simulink model "satellite_dynamics"  (R2025a)
settings: Solver=ode4  StartTime=0.0  StopTime=5400* 5  FixedStep=gyro.Ts  RelTol=1e-6
values from neighbouring files (symbols this model uses):
  altitude = 279e3    (= 279000)    [orbit_params.m]
  G = 6.674e-11    [orbit_params.m]    (also in update_MEKF_new.m = [-eye(3,3), zeros(3,3),zeros(3,3);          zeros(3,3), eye(; update_MEKF_old.m = [-eye(3,3), zeros(3,3);          zeros(3,3), eye(3,3)]; wheel_analysis.m = [ D)
  h_default = h_default + wheel.omega_initial(f) *  wheel.I_II * wheel.axes(:,f)    [orbit_params.m]
  K = convhulln(V)    [wheel_analysis.m]
  m = size(A, 2)    [wheel_analysis.m]
  omega_icrf2b_initial = [-0.3804;-0.2976;0.06] *0    [orbit_params.m]
  P_initial = blkdiag(eye(3) * gyro.sigma_v^2 * 1e4 ,eye(3) * gyro.sigma_u^2 * 1e5)    [orbit_params.m]
  Q_c = blkdiag(eye(3) * gyro.sigma_v^2/2 ,eye(3) * gyro.sigma_u^2/2 )    [orbit_params.m]
  q_icrf2b_initial = q_icrf2b_initial/norm(q_icrf2b_initial)    [orbit_params.m]
  q_initial = q_icrf2b_initial    [orbit_params.m]
  R_k_star = blkdiag(star.sigma_cross^2,star.sigma_cross^2,star.sigma_bore^2) * ((1/3600) * pi/180)^2    [orbit_params.m]
  r_offset = [1;1;5] * 1e-2    [orbit_params.m]
  regulation_kp = regulation.kp    [orbit_params.m]
  s = sign(h_bias)    [min_h.m]
  Ts = 0.1    [orbit_params.m]    (also in untitled2.m = 0.005)
  x_initial = zeros(6,1)    [orbit_params.m]
undefined symbols (not defined in the file or in its folder): DiscIntNeverNeededParam, earth, gyro, Kalman, mag, mag_torque, NEO, regulation, star, sun, tracking, wheel
libraries: utilities x24, simulink_extras x21, aerolibutil x20, dspmathops x19, matrix_library x9, simulink x8, dspstat3 x8, sharedutil x3, aerolibgravity2 x1, eeGeneralControl x1
(part 2 of 2)

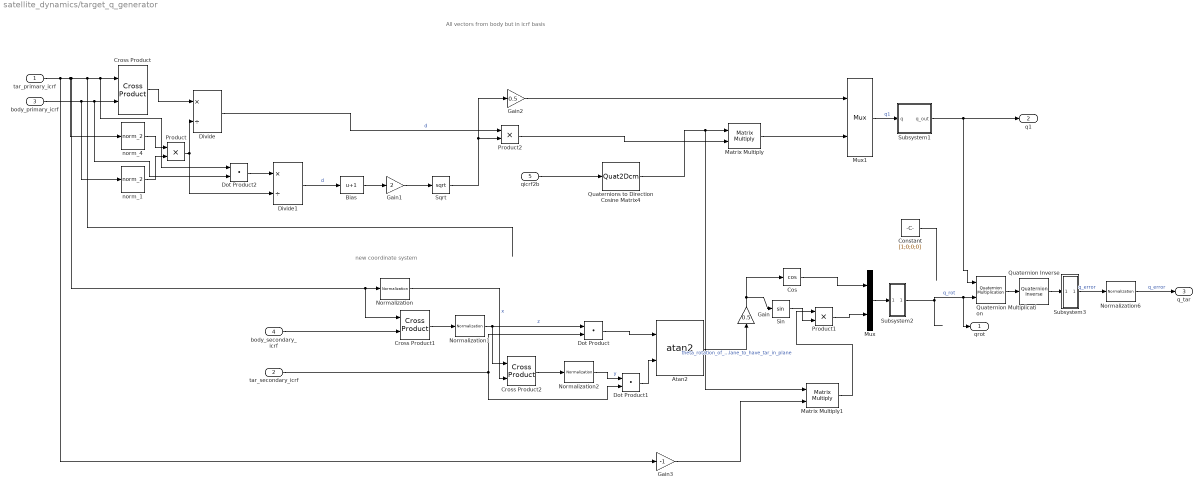
== system satellite_dynamics/target_q_generator ==
  note: new coordinate system
  note: All vectors from body but in icrf basis
  tar_primary_icrf : Inport
  tar_secondary_icrf : Inport  Port=2
  body_primary_icrf : Inport  Port=3
  body_secondary_icrf : Inport  Port=4
  qicrf2b : Inport  Port=5
  Atan2 : Trigonometry  Operator=atan2
  Bias : Bias  Bias=1  SaturateOnIntegerOverflow=off
  Constant : Constant  Value=[1;0;0;0]
  Cos : Trigonometry  Operator=cos
  Cross Product : matrix_library/Cross Product
  Cross Product1 : matrix_library/Cross Product
  Cross Product2 : matrix_library/Cross Product
  Divide : Product  Inputs=*/
  Divide1 : Product  Inputs=*/
  Dot Product : DotProduct  OutDataTypeStr=Inherit: Inherit via internal rule
  Dot Product1 : DotProduct  OutDataTypeStr=Inherit: Inherit via internal rule
  Dot Product2 : DotProduct  OutDataTypeStr=Inherit: Inherit via internal rule
  Gain : Gain  Gain=0.5
  Gain1 : Gain  Gain=2
  Gain2 : Gain  Gain=0.5
  Gain3 : Gain  Gain=-1
  Matrix Multiply : Product  Multiplication=Matrix(*)
  Matrix Multiply1 : Product  Multiplication=Matrix(*)
  Mux : Mux  Inputs=2
  Mux1 : Mux  Inputs=2
  Normalization{,1..2,6} (4 alike) : dspmathops/Normalization  NormType=2-norm  Bias=1e-10  NormOver=Each column  Dimension=1  roundingMode=Floor  overflowMode=off  accumDataTypeStr=Inherit: Same as product output  accumLastDataTypeStr=Inherit: Same as product output  outputDataTypeStr=Inherit: Same as product output  outputMin=[]  outputMax=[]  outputLastDataTypeStr=Inherit: Same as product output
  Product : Product
  Product1 : Product
  Product2 : Product
  Quaternion Inverse : aerolibutil/Quaternion Inverse
  Quaternion Multiplication : aerolibutil/Quaternion Multiplication
  Quaternions to Direction Cosine Matrix4 : Quat2Dcm
  Sin : Trigonometry
  Sqrt : Sqrt
  Subsystem1 : Subsystem
  Subsystem2 : Subsystem
  Subsystem3 : Subsystem
  norm_1 : utilities/norm_2  SystemSampleTime=-1  VariantActivationTime=update diagram  EmptyChoice=off  PassThrough=off  PassThroughVariantControl=(default)  EmptyChoiceVariantControl=(default)  AllowFlexibleInterface=on  Latency=0  AutoFrameSizeCalculation=off
  norm_4 : utilities/norm_2  SystemSampleTime=-1  VariantActivationTime=update diagram  EmptyChoice=off  PassThrough=off  PassThroughVariantControl=(default)  EmptyChoiceVariantControl=(default)  AllowFlexibleInterface=on  Latency=0  AutoFrameSizeCalculation=off
  qrot : Outport
  q1 : Outport  Port=2
  q_tar : Outport  Port=3
  wires:
  tar_primary_icrf/1 -> Gain3/1, Cross Product1/1, Normalization/1, Dot Product2/1, Cross Product/1, norm_4/1
  body_primary_icrf/1 -> norm_1/1, Dot Product2/2, Cross Product/2
  Cross Product/1 -> Divide/1
  norm_4/1 -> Product/1
  norm_1/1 -> Product/2
  Product/1 -> Divide/2, Divide1/2
  Mux1/1 -> Subsystem1/1(q)  "q1"
  Normalization/1 -> Cross Product2/2  "x"
  body_secondary_icrf/1 -> Cross Product1/2
  Cross Product1/1 -> Normalization1/1
  Normalization1/1 -> Cross Product2/1, Dot Product/1  "z"
  Cross Product2/1 -> Normalization2/1
  Normalization2/1 -> Dot Product1/1  "y"
  Atan2/1 -> Gain/1  "theta_rotation_of_plane_to_have_tar_in_plane"
  tar_secondary_icrf/1 -> Dot Product1/2, Dot Product/2
  Dot Product/1 -> Atan2/1
  Dot Product1/1 -> Atan2/2
  Mux/1 -> Subsystem2/1(q)
  Cos/1 -> Mux/1
  Gain/1 -> Sin/1, Cos/1
  Sin/1 -> Product1/2
  Product1/1 -> Mux/2
  Quaternion Multiplication/1 -> Quaternion Inverse/1
  Divide/1 -> Product2/1  "d"
  Dot Product2/1 -> Divide1/1
  Divide1/1 -> Bias/1  "d"
  Bias/1 -> Gain1/1
  Gain1/1 -> Sqrt/1
  Gain2/1 -> Mux1/1
  Sqrt/1 -> Product2/2, Gain2/1
  Product2/1 -> Matrix Multiply/2
  Subsystem1/1(q_out) -> Quaternion Multiplication/1, q1/1
  Subsystem2/1(q_out) -> qrot/1, Quaternion Multiplication/2  "q_rot"
  Subsystem3/1(q_out) -> Normalization6/1  "q_error"
  Constant/1 -> ?
  qicrf2b/1 -> Quaternions to Direction Cosine Matrix4/1
  Quaternions to Direction Cosine Matrix4/1 -> Matrix Multiply1/1, Matrix Multiply/1
  Matrix Multiply/1 -> Mux1/2
  Gain3/1 -> Matrix Multiply1/2
  Matrix Multiply1/1 -> Product1/1
  Normalization6/1 -> q_tar/1  "q_error"
  Quaternion Inverse/1 -> Subsystem3/1(q)

== system satellite_dynamics/wheel_controller ==
  qicrf2b : Inport
  qicrf2lvlh : Inport  Port=2
  Enable : EnablePort
  LVLH_pointing : Subsystem
  PID_controller : Subsystem
  wheel_torque : Outport
  wires:
  LVLH_pointing/1(q_error) -> PID_controller/1(q_error)  "stad"
  PID_controller/1(wheel_torque) -> wheel_torque/1  "wheel_torque"
  qicrf2b/1 -> LVLH_pointing/1(qicrf2b)
  qicrf2lvlh/1 -> LVLH_pointing/2(qicrf2lvlh)

== system satellite_dynamics/wheels_dynamics ==
  wheel_torques : Inport
  satellite_body_omega_dot : Inport  Port=2
  Add : Sum  Inputs=++++
  Add1 : Sum  Inputs=++++
  Demux : Demux
  wheel_dynamics : utilities/wheel_dynamics  wheel=wheel  no=1
  wheel_dynamics1 : utilities/wheel_dynamics  wheel=wheel  no=2
  wheel_dynamics2 : utilities/wheel_dynamics  wheel=wheel  no=3
  wheel_dynamics3 : utilities/wheel_dynamics  wheel=wheel  no=4
  body_torque : Outport
  angular_momentum_body : Outport  Port=2
  wires:
  wheel_torques/1 -> Demux/1
  Demux/1 -> wheel_dynamics/1
  Demux/2 -> wheel_dynamics1/1
  Demux/3 -> wheel_dynamics2/1
  Demux/4 -> wheel_dynamics3/1
  wheel_dynamics/1 -> Add1/1
  wheel_dynamics/4 -> Add/1
  wheel_dynamics1/4 -> Add/2
  wheel_dynamics2/4 -> Add/3
  wheel_dynamics3/4 -> Add/4
  Add/1 -> body_torque/1
  wheel_dynamics1/1 -> Add1/2
  wheel_dynamics2/1 -> Add1/3
  wheel_dynamics3/1 -> Add1/4
  wheel_dynamics/2 -> ?
  wheel_dynamics/3 -> ?
  wheel_dynamics1/2 -> ?
  wheel_dynamics1/3 -> ?
  wheel_dynamics2/2 -> ?
  wheel_dynamics2/3 -> ?
  wheel_dynamics3/2 -> ?
  wheel_dynamics3/3 -> ?
  satellite_body_omega_dot/1 -> wheel_dynamics/2, wheel_dynamics1/2, wheel_dynamics2/2, wheel_dynamics3/2
  Add1/1 -> angular_momentum_body/1

== system satellite_dynamics/Feedforward_torque_legacy/w_ref ==
  Xicrf : Inport
  Vicrf : Inport  Port=2
  Cross Product : matrix_library/Cross Product
  Gain : Gain  Gain=sqrt(G * earth.Mass/(earth.R + altitude)^3)
  Normalization1 : dspmathops/Normalization  NormType=2-norm  Bias=1e-10  NormOver=Each column  Dimension=1  roundingMode=Floor  overflowMode=off  accumDataTypeStr=Inherit: Same as product output  accumLastDataTypeStr=Inherit: Same as product output  outputDataTypeStr=Inherit: Same as product output  outputMin=[]  outputMax=[]  outputLastDataTypeStr=Inherit: Same as product output
  Normalization2 : dspmathops/Normalization  NormType=2-norm  Bias=1e-10  NormOver=Each column  Dimension=1  roundingMode=Floor  overflowMode=off  accumDataTypeStr=Inherit: Same as product output  accumLastDataTypeStr=Inherit: Same as product output  outputDataTypeStr=Inherit: Same as product output  outputMin=[]  outputMax=[]  outputLastDataTypeStr=Inherit: Same as product output
  ref : Outport
  wires:
  Xicrf/1 -> Normalization1/1
  Vicrf/1 -> Normalization2/1
  Normalization1/1 -> Cross Product/1
  Normalization2/1 -> Cross Product/2
  Cross Product/1 -> Gain/1  "axis_to_rotate"
  Gain/1 -> ref/1

== system satellite_dynamics/Subsystem6/Subsystem1 ==
  q : Inport
  Compare To Constant : simulink/Logic and Bit Operations/Compare To Constant  relop=<  const=0  OutDataTypeStr=boolean
  Gain : Gain  Gain=-1
  Selector : Selector  InputPortWidth=4  IndexOptions=Index vector (dialog)  Indices=[1]  OutputSizes=1
  Switch : Switch  Criteria=u2 > Threshold  SaturateOnIntegerOverflow=off  InputSameDT=off
  q_out : Outport
  wires:
  q/1 -> Gain/1, Selector/1, Switch/3
  Switch/1 -> q_out/1
  Selector/1 -> Compare To Constant/1
  Compare To Constant/1 -> Switch/2
  Gain/1 -> Switch/1

== system satellite_dynamics/target_q_generator/Subsystem1 ==
  q : Inport
  Compare To Constant : simulink/Logic and Bit Operations/Compare To Constant  relop=<  const=0  OutDataTypeStr=boolean
  Gain : Gain  Gain=-1
  Selector : Selector  InputPortWidth=4  IndexOptions=Index vector (dialog)  Indices=[1]  OutputSizes=1
  Switch : Switch  Criteria=u2 > Threshold  SaturateOnIntegerOverflow=off  InputSameDT=off
  q_out : Outport
  wires:
  q/1 -> Gain/1, Selector/1, Switch/3
  Switch/1 -> q_out/1
  Selector/1 -> Compare To Constant/1
  Compare To Constant/1 -> Switch/2
  Gain/1 -> Switch/1

== system satellite_dynamics/target_q_generator/Subsystem2 ==
  q : Inport
  Compare To Constant : simulink/Logic and Bit Operations/Compare To Constant  relop=<  const=0  OutDataTypeStr=boolean
  Gain : Gain  Gain=-1
  Selector : Selector  InputPortWidth=4  IndexOptions=Index vector (dialog)  Indices=[1]  OutputSizes=1
  Switch : Switch  Criteria=u2 > Threshold  SaturateOnIntegerOverflow=off  InputSameDT=off
  q_out : Outport
  wires:
  q/1 -> Gain/1, Selector/1, Switch/3
  Switch/1 -> q_out/1
  Selector/1 -> Compare To Constant/1
  Compare To Constant/1 -> Switch/2
  Gain/1 -> Switch/1

== system satellite_dynamics/target_q_generator/Subsystem3 ==
  q : Inport
  Compare To Constant : simulink/Logic and Bit Operations/Compare To Constant  relop=<  const=0  OutDataTypeStr=boolean
  Gain : Gain  Gain=-1
  Selector : Selector  InputPortWidth=4  IndexOptions=Index vector (dialog)  Indices=[1]  OutputSizes=1
  Switch : Switch  Criteria=u2 > Threshold  SaturateOnIntegerOverflow=off  InputSameDT=off
  q_out : Outport
  wires:
  q/1 -> Gain/1, Selector/1, Switch/3
  Switch/1 -> q_out/1
  Selector/1 -> Compare To Constant/1
  Compare To Constant/1 -> Switch/2
  Gain/1 -> Switch/1

== system satellite_dynamics/wheel_controller/LVLH_pointing ==
  qicrf2b : Inport
  qicrf2lvlh : Inport  Port=2
  Normalization : dspmathops/Normalization  NormType=2-norm  Bias=1e-10  NormOver=Each column  Dimension=1  roundingMode=Floor  overflowMode=off  accumDataTypeStr=Inherit: Same as product output  accumLastDataTypeStr=Inherit: Same as product output  outputDataTypeStr=Inherit: Same as product output  outputMin=[]  outputMax=[]  outputLastDataTypeStr=Inherit: Same as product output
  Normalization1 : dspmathops/Normalization  NormType=2-norm  Bias=1e-10  NormOver=Each column  Dimension=1  roundingMode=Floor  overflowMode=off  accumDataTypeStr=Inherit: Same as product output  accumLastDataTypeStr=Inherit: Same as product output  outputDataTypeStr=Inherit: Same as product output  outputMin=[]  outputMax=[]  outputLastDataTypeStr=Inherit: Same as product output
  Quaternion Inverse : aerolibutil/Quaternion Inverse
  Quaternion Multiplication : aerolibutil/Quaternion Multiplication
  Quaternion Normalize : sharedutil/Quaternion Normalize  aMode=aMode
  Subsystem1 : Subsystem
  Terminator : Terminator
  vector_magnitude : utilities/vector_magnitude
  q_error : Outport
  wires:
  qicrf2b/1 -> Normalization/1
  Quaternion Multiplication/1 -> vector_magnitude/1, Quaternion Normalize/1
  Normalization/1 -> Quaternion Inverse/1
  Quaternion Inverse/1 -> Quaternion Multiplication/1
  vector_magnitude/1 -> Terminator/1
  Normalization1/1 -> Quaternion Multiplication/2
  Quaternion Normalize/1 -> Subsystem1/1(q)
  qicrf2lvlh/1 -> Normalization1/1
  Subsystem1/1(q_out) -> q_error/1  "q_error"

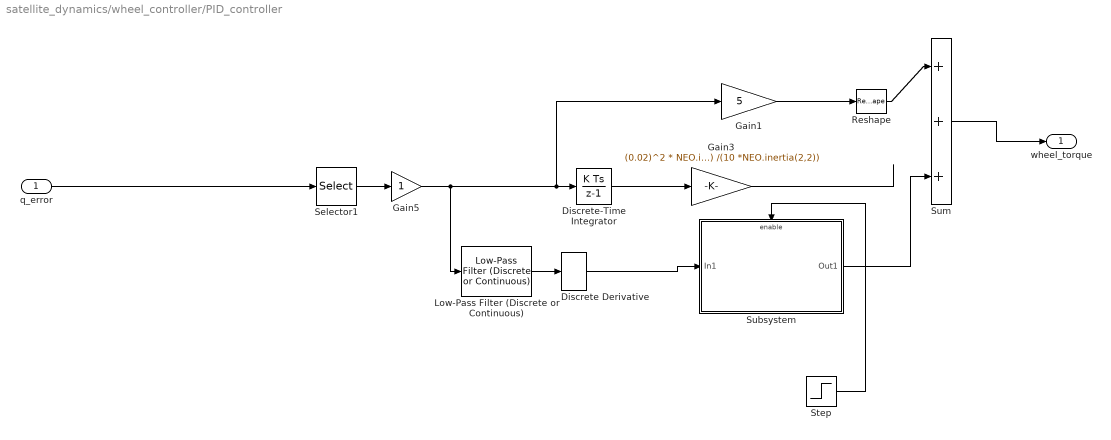
== system satellite_dynamics/wheel_controller/PID_controller ==
  q_error : Inport
  Discrete Derivative : simulink/Discrete/Discrete Derivative  gainval=1.0  ICPrevScaledInput=0.0  OutMin=[]  OutMax=[]  OutDataType=fixdt(1, 16)  OutScaling=2^-10  DoSatur=off
  Discrete-Time Integrator : DiscreteIntegrator  SampleTime=-1  ICPrevOutput=DiscIntNeverNeededParam  ICPrevScaledInput=DiscIntNeverNeededParam
  Gain1 : Gain  Gain=5
  Gain3 : Gain  Gain="(0.02)^2 * NEO.inertia(2,2) * 2 * 0.7 * 0.02 *  NEO.inertia(2,2) /(10 *NEO.inertia(2,2))"
  Gain5 : Gain
  Low-Pass Filter (Discrete or Continuous) : eeGeneralControl/Low-Pass Filter (Discrete or Continuous)  K=1  T=1  B=inf  A=-inf  init_option=Inherited from block input  x0=0  Ts=-1
  Reshape : Reshape
  Selector1 : Selector  InputPortWidth=4  IndexOptions=Index vector (dialog)  Indices=[2:4]  OutputSizes=1
  Step : Step  Time=5  SampleTime=0
  Subsystem : Subsystem
  Sum : Sum  Inputs=|+++
  wheel_torque : Outport  PortDimensions=[3,1]
  wires:
  Gain3/1 -> ?
  Gain5/1 -> Low-Pass Filter (Discrete or Continuous)/1, Discrete-Time Integrator/1, Gain1/1
  Gain1/1 -> Reshape/1
  q_error/1 -> Selector1/1
  Discrete-Time Integrator/1 -> Gain3/1
  Selector1/1 -> Gain5/1
  Reshape/1 -> Sum/1
  Sum/1 -> wheel_torque/1
  Low-Pass Filter (Discrete or Continuous)/1 -> Discrete Derivative/1
  Discrete Derivative/1 -> Subsystem/1(In1)
  Subsystem/1(Out1) -> Sum/3
  Step/1 -> Subsystem/Enable

== system satellite_dynamics/wheel_controller/LVLH_pointing/Subsystem1 ==
  q : Inport
  Compare To Constant : simulink/Logic and Bit Operations/Compare To Constant  relop=<  const=0  OutDataTypeStr=boolean
  Gain : Gain  Gain=-1
  Selector : Selector  InputPortWidth=4  IndexOptions=Index vector (dialog)  Indices=[1]  OutputSizes=1
  Switch : Switch  Criteria=u2 > Threshold  SaturateOnIntegerOverflow=off  InputSameDT=off
  q_out : Outport
  wires:
  q/1 -> Gain/1, Selector/1, Switch/3
  Switch/1 -> q_out/1
  Selector/1 -> Compare To Constant/1
  Compare To Constant/1 -> Switch/2
  Gain/1 -> Switch/1

== system satellite_dynamics/wheel_controller/PID_controller/Subsystem ==
  In1 : Inport
  Enable : EnablePort
  Gain2 : Gain  Gain="2 * 0.7 * 0.02 *  NEO.inertia(2,2) * 10"
  Out1 : Outport
  wires:
  Gain2/1 -> Out1/1
  In1/1 -> Gain2/1

== matlab function satellite_dynamics/average_angle_knowledge_error1/MATLAB Function ==
  data: u input; y output
function y = fcn(u)

if u < 0
    y = u + 180;
else
    y = u;
end

== matlab function satellite_dynamics/earth_tracking_controller ==
  data: q_icrf2lvlh input; torque output; q_icrf2b input; X_icrf input; V_icrf input; V_icrf_dot input; omega_b input; omega_c output; NEO parameter; tracking parameter; dq input; dA output; dq_int input
function [torque,omega_c,dA] = fcn(q_icrf2lvlh,q_icrf2b,X_icrf,V_icrf,V_icrf_dot,omega_b, NEO, tracking,dq, dq_int)


dcm_icrf2lvlh = quat2dcm(q_icrf2lvlh');
dcm_lvlh2icrf = dcm_icrf2lvlh';
dcm_icrf2b = quat2dcm(q_icrf2b');


omega_c = [0;-norm(cross(X_icrf,V_icrf))/ (norm(X_icrf)^2)  ; norm(X_icrf) * (dcm_lvlh2icrf(:,2)' * V_icrf_dot) / norm(cross(X_icrf,V_icrf))  ];  %%% lvlh angular vel wrt inertial frame expressed in lvlh coordiantew

omega_c_dot = [0;0;0]; %% zero for now


dA = dcm_icrf2b * dcm_icrf2lvlh';
dw = omega_b - dA * omega_c;




torque = skew_sym_mat(dA * omega_c) * NEO.inertia * dA * omega_c + NEO.inertia * dA * omega_c_dot - tracking.kp .* dq(2:4) - tracking.kd .* dw  - dq_int .* [1;1;1] * 1e-3 ;

== matlab function satellite_dynamics/regulating_controller ==
  data: q_icrf2tar input; torque output; q_icrf2b input; hwheelsbody input; regulation parameter; omega_b input; dq output; regulation_kp parameter; K parameter
function [torque,dq]  = fcn(q_icrf2tar,q_icrf2b,hwheelsbody, regulation,omega_b, regulation_kp, K)


dq = quatmultiply_olgu(q_icrf2b',quatinv(q_icrf2tar'))';

torque_eq =  - regulation_kp .* sign(dq(1)) .* dq(2:4) - regulation.kd .* (1 - dq(2:4)' * dq(2:4)) .* omega_b;

% theta_err = 2 * sign(dq(1)) .* dq(2:4);
% omega_err = omega_b;
% 
% x = [theta_err;
%      omega_err];
% 
% torque_eq  = -K * x;

% torque_eq =  - regulation.kp * sign(dq(1)) * dq(2:4) - regulation.kd * omega_b;


%%% minus to have it be the torque demanded on the spacecraft rather than
%%% the wheels
torque = -(-torque_eq - skew_sym_mat(omega_b) * hwheelsbody);

== matlab function satellite_dynamics/MATLAB Function ==
  data: angle_deg input; quat output; vector input
function quat = fcn(angle_deg,vector)

quat = [cosd(angle_deg/2);vector/norm(vector) .* sind(angle_deg/2)];
quat = quat/norm(quat);

== matlab function satellite_dynamics/MEKF ==
  data: omega_icrf2b_gyro input; q_k_k output; q_icrf2b_star input size=[4,1]; star_valid input; sun_vectors input; sun_valid input; mag_XYZ_icrf_model input; mag_XYZ_body_meas input; mag_valid input; sat2sun_icrf input; x_initial parameter; q_initial parameter; Kalman parameter; P_initial parameter; x_k_k output; Q_c parameter; star parameter; R_k_star parameter; sun parameter; mag parameter; gyro parameter
function [q_k_k,x_k_k] = update_MEKF(omega_icrf2b_gyro,q_icrf2b_star,star_valid,sun_vectors,sun_valid, mag_XYZ_icrf_model,mag_XYZ_body_meas,mag_valid, sat2sun_icrf,x_initial, q_initial, Kalman, P_initial, Q_c, star, R_k_star, sun, mag, gyro)


persistent q_k_k_state P_k_k_state x_k_k_state tick

if isempty(q_k_k_state) 
    x_k_k_state = x_initial;   %%% error state
    q_k_k_state = q_initial; %%%%% initial quaternion
    P_k_k_state = P_initial;
    tick = uint64(0);
end
x_k1_k1 = x_k_k_state;
q_k1_k1 = q_k_k_state;
P_k1_k1 = P_k_k_state;


%%%%%%%%
% x = [a;bias]
omega_icrf2b_gyro_unbiased = omega_icrf2b_gyro - x_k1_k1(4:6);


%%%%% Omega matrix
w_cross = [  0   -omega_icrf2b_gyro_unbiased(3)   omega_icrf2b_gyro_unbiased(2);
            omega_icrf2b_gyro_unbiased(3)    0   -omega_icrf2b_gyro_unbiased(1);
           -omega_icrf2b_gyro_unbiased(2)   omega_icrf2b_gyro_unbiased(1)    0 ];
w_mat = [0        -omega_icrf2b_gyro_unbiased';
         omega_icrf2b_gyro_unbiased    -w_cross];




%%% Get a priori quaternion
% q_icrf2b_dot = 0.5 * w_mat * q_k1_k1;
% x_k_k1 = [zeros(3,1);x_k1_k1(4:6)];
% 
% q_k_k1 = q_k1_k1 + q_icrf2b_dot * Kalman.Ts;

%% NEW FROM BOOK
d_theta = 0.5 * norm(omega_icrf2b_gyro_unbiased) * Kalman.Ts;
PHI_k = sin(d_theta) * omega_icrf2b_gyro_unbiased/norm(omega_icrf2b_gyro_unbiased);

OMEGA_k = [cos(d_theta) * eye(3) - skew_sym_mat(PHI_k), PHI_k;
    -PHI_k', cos(d_theta)];

q_k_k1_convention = OMEGA_k * [q_k1_k1(2:4);q_k1_k1(1)];
q_k_k1 = [q_k_k1_convention(4);q_k_k1_convention(1:3)];
x_k_k1 = [zeros(3,1);x_k1_k1(4:6)];




q_k_k1 = q_k_k1 / norm(q_k_k1);
    %%%get continious model
    
    % F = [-w_cross,  -eye(3,3)  ; ...
    %     zeros(3,3),  zeros(3,3)];   %%%% skew symetric w cross
    
    G = [-eye(3,3), zeros(3,3); ...
        zeros(3,3), eye(3,3)];
    
    
    
    %%%
    %%old old
    % % % % Q_c = [eye(6,6)] * 1e-6;
    % % % % Q_k = G * Q_c * G' * Kalman.Ts;
    % % % % Q_k = Q_c;
    % old
%     Phi_k = eye(6,6) + F * Kalman.Ts;
%     % Q_k = [gyro_sigma_rad_v^2*Kalman.Ts/2 + 1/3 * gyro_sigma_rad_u^2/2 * Kalman.Ts * eye(3),-(0.5 * gyro_sigma_rad_u^2/2 * Kalman.Ts^2) * eye(3);-(0.5*gyro_sigma_rad_u^2/2 * Kalman.Ts^2) * eye(3),(gyro_sigma_rad_u^2/2 * Kalman.Ts  * eye(3) )];
% Q_k = [(gyro_sigma_rad_v^2*Kalman.Ts/2 + 1/3 * gyro_sigma_rad_u^2/2 * Kalman.Ts^3) * eye(3),-(0.5 * gyro_sigma_rad_u^2/2 * Kalman.Ts^2) * eye(3); ...
%     -(0.5*gyro_sigma_rad_u^2/2 * Kalman.Ts^2) * eye(3),(gyro_sigma_rad_u^2/2 * Kalman.Ts  * eye(3) )];
%     P_k_k1 = Phi_k * P_k1_k1 * Phi_k' + Q_k;
%% NEW FROM BOOK
gyro_sigma_rad_u = gyro.sigma_u * pi/180 / sqrt(Kalman.Ts/gyro.Ts) / sqrt(2);  %% taking into account two gyros averaged
gyro_sigma_rad_v = gyro.sigma_v * pi/180 / sqrt(Kalman.Ts/gyro.Ts) / sqrt(2);

Q_k = [(gyro_sigma_rad_v^2*Kalman.Ts + 1/3 * gyro_sigma_rad_u^2 * Kalman.Ts^3) * eye(3),-(0.5 * gyro_sigma_rad_u^2/2 * Kalman.Ts^2) * eye(3); ...
    -(0.5*gyro_sigma_rad_u^2/2 * Kalman.Ts^2) * eye(3),(gyro_sigma_rad_u^2/2 * Kalman.Ts  * eye(3) )];

Phi_k_11 = eye(3) - w_cross * sin(norm(omega_icrf2b_gyro_unbiased * Kalman.Ts))/norm(omega_icrf2b_gyro_unbiased) ...
    + w_cross * w_cross * (1 - cos(norm(omega_icrf2b_gyro_unbiased) * Kalman.Ts))/norm(omega_icrf2b_gyro_unbiased)^2;
Phi_k_12 = w_cross * (1 - cos(norm(omega_icrf2b_gyro_unbiased) * Kalman.Ts))/norm(omega_icrf2b_gyro_unbiased)^2 - eye(3) * Kalman.Ts ...
    -w_cross * w_cross * (norm(omega_icrf2b_gyro_unbiased) * Kalman.Ts - sin(norm(omega_icrf2b_gyro_unbiased) * Kalman.Ts))/norm(omega_icrf2b_gyro_unbiased)^3;

Phi_k = [Phi_k_11,Phi_k_12;
    zeros(3,3),eye(3,3)];
P_k_k1 = Phi_k * P_k1_k1 * Phi_k' + G * Q_k * G';

if star_valid && mod(tick,uint64(star.Ts/Kalman.Ts)) == uint64(0)
    %%%%%%%%%% Star

    
    
    %% measurment matrix simple   % star tracket
    H_k = [eye(3,3),zeros(3,3)];
    
    
    %%%kalman gain and mearuement error
    % R_k = eye(3,3) * 1e-6;
    
    R_k = star.dcm_b2star' * R_k_star * star.dcm_b2star;
    K_k = P_k_k1*H_k'/(H_k*P_k_k1*H_k' + R_k);
    
    
    dq_star = quatmultiply(quatinv(q_k_k1'),q_icrf2b_star')';
    if dq_star(1) < 0
        dq_star = -dq_star;
    end
    x_star = 2*[dq_star(2:4)];
    
    x_k_k = x_k_k1 + K_k * (x_star - H_k * x_k_k1);
    % P_k_k = (eye(6,6) - K_k * H_k)*P_k_k1;    %%% changet to Joseph form
    P_k_k = (eye(6,6) - K_k * H_k) * P_k_k1 * (eye(6,6) - K_k * H_k)' + K_k * R_k * K_k';


    %% get quat
    dq = [1;0.5 * x_k_k(1:3)];
    dq = dq/norm(dq);
    
    q_k_k = quatmultiply(q_k_k1',dq')';
    q_k_k = q_k_k/norm(q_k_k);
    
    x_k_k(1:3) = 0;
    

    %%Covar reset if wanted from file:///C:/Users/OlguPilav/Downloads/Covariance_Reset_JGCD_2023.pdf
    % qhat_13 = dq(2:4);   % vector part of the injected correction quaternion
    % 
    % S = [           0   -qhat_13(3)   qhat_13(2);
    %       qhat_13(3)             0   -qhat_13(1);
    %      -qhat_13(2)    qhat_13(1)            0 ];
    % 
    % Gamma_q = (eye(3) + S*S)/sqrt(1 - qhat_13'*qhat_13) - S;
    % 
    % G_reset = eye(6);
    % G_reset(1:3,1:3) = Gamma_q;
    % 
    % P_k_k = G_reset * P_k_k * G_reset';
    % P_k_k = 0.5*(P_k_k + P_k_k');
else
    x_k_k = x_k_k1;
    P_k_k = P_k_k1;

    dq = [1;0.5 * x_k_k(1:3)];
    dq = dq/norm(dq);
    
    q_k_k = quatmultiply(q_k_k1',dq')';
    q_k_k = q_k_k/norm(q_k_k);
    x_k_k(1:3) = 0;

end
%%%%%%% star tracker end
% disp(mod(tick,uint64(sun.Ts/Kalman.Ts)))
% disp(tick)
if any(sun_valid) && mod(tick,uint64(sun.Ts/Kalman.Ts)) == uint64(0) && ~star_valid
    %%%%%%%%%% prev  mag_XYZ_icrf_model,mag_XYZ_body_meas,mag_valid
    P_k_k1 = P_k_k;
    x_k_k1 = x_k_k;
    q_k_k1 = q_k_k;

        %%%valid FSS no
    FSS_no = sum(sun_valid == 1);
    sun_vectors_valid = sun_vectors(:,:,sun_valid);

    %% normalise
    sat2sun_icrf = sat2sun_icrf/norm(sat2sun_icrf);

    for kk = 1:FSS_no
        sun_vectors_valid(:,:,kk) = sun_vectors_valid(:,:,kk)/norm(sun_vectors_valid(:,:,kk));
    end
    




    %% get current rotation matrix
    q_k_k1;
    dcm_icrf2b = quat2dcm(q_k_k1');

    %%%kalman gain and mearuement error    
    R_k_sun = eye(FSS_no*3) * sun.sigma^2;



    % R_k_sun_one = 10000000 *sun.sigma^2 * (eye(3) - sat2sun_body*sat2sun_body') + 10000000 * sun.sigma^2 * (sat2sun_body*sat2sun_body');
    % R_k_sun = kron(eye(FSS_no), R_k_sun_one);

    sat2sun_body = dcm_icrf2b * sat2sun_icrf;
    sat2sun_body_skew = [0, -sat2sun_body(3), sat2sun_body(2);
        sat2sun_body(3), 0, -sat2sun_body(1);
        -sat2sun_body(2), sat2sun_body(1), 0];

    H_k_row = [sat2sun_body_skew,zeros(3,3)];
    H_k = repmat(H_k_row,FSS_no,1);


    K_k = P_k_k1*H_k'/(H_k*P_k_k1*H_k' + R_k_sun);

    % sun_vectors_valid_body = pagemtimes(dcm_icrf2b,sun_vectors_valid);
    y_k = reshape(sun_vectors_valid, [], 1);%%% measurment in body frame stacked already in body pay attention

    h_x_k = repmat(sat2sun_body,FSS_no,1);


    x_k_k = x_k_k1 + K_k * (y_k - h_x_k);
    % 
    P_k_k = (eye(6,6) - K_k * H_k) * P_k_k1 * (eye(6,6) - K_k * H_k)' + K_k * R_k_sun * K_k';

    %% get quat
    dq = [1;0.5 * x_k_k(1:3)];
    dq = dq/norm(dq);
    
    q_k_k = quatmultiply(q_k_k1',dq')';
    q_k_k = q_k_k/norm(q_k_k);
    
    x_k_k(1:3) = 0;

    % disp('sun')
    % disp(tick)
    % disp('sun')
else
    % x_k_k = x_k_k;
    % P_k_k = P_k_k;
end
% 
% %%%%%% sun sensor start
if mag_valid && mod(tick,uint64(mag.Ts/Kalman.Ts)) == uint64(0) && ~star_valid
    %%%%%%%%%% prev  mag_XYZ_icrf_model,mag_XYZ_body_meas,mag_valid
    P_k_k1 = P_k_k;
    x_k_k1 = x_k_k;
    q_k_k1 = q_k_k;

    %% normalise
    mag_XYZ_icrf_model = mag_XYZ_icrf_model/norm(mag_XYZ_icrf_model);


    R_k_mag = mag.R_k/norm(mag_XYZ_body_meas)^2;
    % R_k_mag = mag.R_k;

    mag_XYZ_body_meas = mag_XYZ_body_meas/norm(mag_XYZ_body_meas);


    


    %% get current rotation matrix
    q_k_k1;
    dcm_icrf2b = quat2dcm(q_k_k1');


    %%%kalman gain and mearuement error    
    


    mag_XYZ_body_model = dcm_icrf2b * mag_XYZ_icrf_model;

    % R_k_sun_one = 10000000 *sun.sigma^2 * (eye(3) - sat2sun_body*sat2sun_body') + 10000000 * sun.sigma^2 * (sat2sun_body*sat2sun_body');
    % R_k_sun = kron(eye(FSS_no), R_k_sun_one);

    mag_XYZ_body_model_skew = [0, -mag_XYZ_body_model(3), mag_XYZ_body_model(2);
        mag_XYZ_body_model(3), 0, -mag_XYZ_body_model(1);
        -mag_XYZ_body_model(2), mag_XYZ_body_model(1), 0];

    H_k_row = [mag_XYZ_body_model_skew,zeros(3,3)];
    H_k = H_k_row;


    K_k = P_k_k1*H_k'/(H_k*P_k_k1*H_k' + R_k_mag);

    % sun_vectors_valid_body = pagemtimes(dcm_icrf2b,sun_vectors_valid);
    y_k = mag_XYZ_body_meas;

    h_x_k = mag_XYZ_body_model;


    x_k_k = x_k_k1 + K_k * (y_k - h_x_k);
    % 
    P_k_k = (eye(6,6) - K_k * H_k) * P_k_k1 * (eye(6,6) - K_k * H_k)' + K_k * R_k_mag * K_k';

    %% get quat
    dq = [1;0.5 * x_k_k(1:3)];
    dq = dq/norm(dq);

    q_k_k = quatmultiply(q_k_k1',dq')';
    q_k_k = q_k_k/norm(q_k_k);

    x_k_k(1:3) = 0;

    % 
    % disp('mag')
    % disp(tick)
    % disp('mag')
else
    % x_k_k = x_k_k;
    % P_k_k = P_k_k;
end


% dq = [1;0.5 * x_k_k(1:3)];
% dq = dq/norm(dq);
% 
% q_k_k = quatmultiply(q_k_k1',dq')';
% q_k_k = q_k_k/norm(q_k_k);
% 
% 
% 
% 
% x_k_k(1:3) = 0;

q_k_k_state = q_k_k;
x_k_k_state = x_k_k;
P_k_k_state = P_k_k;
tick = tick + 1;

== matlab function satellite_dynamics/olgus_dynamics/MATLAB Function ==
  data: Mb input size=[3,1]; q_icrf2b_out output size=[4,1]; omega_icrf2b input size=[3,1]; Imom input; q_icrf2b input size=[4,1]; omega_icrf2b_out output size=[3,1]; Ts parameter; h_wheels_body input; omega_icrf2b_out_dot output
function [q_icrf2b_out,omega_icrf2b_out,omega_icrf2b_out_dot] = fcn(Mb,omega_icrf2b,Imom,q_icrf2b, Ts, h_wheels_body)




% 
k1 =  Imom \ (Mb - cross(omega_icrf2b, Imom*omega_icrf2b - h_wheels_body));

omega2 = omega_icrf2b + 0.5*Ts*k1;
k2 =  Imom \ (Mb - cross(omega2, Imom*omega2 - h_wheels_body));

omega3 = omega_icrf2b + 0.5*Ts*k2;
k3 =  Imom \ (Mb - cross(omega3, Imom*omega3 - h_wheels_body));

omega4 = omega_icrf2b + Ts*k3;
k4 =  Imom \ (Mb - cross(omega4, Imom*omega4 - h_wheels_body));

omega_icrf2b_out = omega_icrf2b + (Ts/6) * (k1 + 2*k2 + 2*k3 + k4);
% 
omega_icrf2b_out_dot = (1/6) * (k1 + 2*k2 + 2*k3 + k4);


% 
% omega_icrf2b_dot = Imom \ (Mb - cross(omega_icrf2b, Imom*omega_icrf2b));
% 
% omega_icrf2b_out_mid = omega_icrf2b + omega_icrf2b_dot * Ts/2;
% 
% omega_icrf2b_dot = Imom \ (Mb - cross(omega_icrf2b_out_mid, Imom*omega_icrf2b_out_mid));
% 
% omega_icrf2b_out = omega_icrf2b + omega_icrf2b_dot * Ts;



%w_mat = [0 omega_icrf2b(1) omega_icrf2b(2) omega_icrf2b(3); ...
%    -omega_icrf2b(1) 0 -omega_icrf2b(3) omega_icrf2b(2); ...
 %   -omega_icrf2b(2) omega_icrf2b(3) 0 -omega_icrf2b(1); ...
 %   -omega_icrf2b(3) -omega_icrf2b(2) omega_icrf2b(1) 0];


omega_icrf2b = (omega_icrf2b + omega_icrf2b_out)/2;
w_cross = [  0   -omega_icrf2b(3)   omega_icrf2b(2);
            omega_icrf2b(3)    0   -omega_icrf2b(1);
           -omega_icrf2b(2)   omega_icrf2b(1)    0 ];

w_mat = [0        -omega_icrf2b';
         omega_icrf2b    -w_cross];


q_icrf2b_dot = 0.5 * w_mat * q_icrf2b;
q_icrf2b_out = q_icrf2b + q_icrf2b_dot * Ts;
% 
% 

% 
% omega_icrf2b_avg = (omega_icrf2b + omega_icrf2b_out)/2;
% 
% disp("omega_icrf2b_avg")
% disp(omega_icrf2b_avg)
% theta = norm(omega_icrf2b_avg * Ts);
% 
% 
% u = omega_icrf2b_avg * Ts/(theta + 1e-6);
% 
% disp('u')
% disp(u)
% 
% dq = [cos(theta/2);sin(theta/2) * u];
% disp("dq")
% disp(dq)
% 
% q_icrf2b_out = quatmultiply(q_icrf2b',dq')';
% disp("q_icrf2b_out1")
% disp(q_icrf2b_out)

q_icrf2b_out = q_icrf2b_out / norm(q_icrf2b_out);

== matlab function satellite_dynamics/magnetic_field_slow/MATLAB Function ==
  data: lat input; ned2ecef output; long input
function ned2ecef = fcn(lat,long)


ned2ecef = [-sind(lat) * cosd(long),-sind(lat)*sind(long),cosd(lat);
    -sind(long),cosd(long),0;
    -cosd(lat)*cosd(long),-cosd(lat)*sind(long),sind(lat)]';

end

== matlab function satellite_dynamics/average_angle_knowledge_error/MATLAB Function ==
  data: u input; y output
function y = fcn(u)

if u < 0
    y = u + 180;
else
    y = u;
end

== matlab function satellite_dynamics/MATLAB Function1 ==
  data: b1 input; y output; b2 input; sun parameter; mag parameter
function y = fcn(b1,b2, sun, mag)


b1 = b1/norm(b1);
sigma_1 = sun.sigma; %% rad



sigma_2 = mag.sigma/norm(b2);
b2 = b2/norm(b2);

P_sigma_sigma = (sigma_2 ^2 * b1 * b1' + sigma_1^2 * b2 * b2') / norm(cross(b1,b2))^2 + sigma_1^2 * sigma_2^2 * cross(b1,b2) * cross(b1,b2)' / (sigma_1^2 + sigma_2^2) /norm(cross(b1,b2))^2;

a = sqrt((P_sigma_sigma(1,1))) * 180/pi * 3600;
b = sqrt((P_sigma_sigma(2,2))) * 180/pi * 3600;
c = sqrt((P_sigma_sigma(3,3))) * 180/pi * 3600;

y = [a;b;c];

== matlab function satellite_dynamics/olgus_dynamics/MATLAB Function1 ==
  data: q_icrf2b_out output size=[4,1]; omega_icrf2b input size=[3,1]; q_icrf2b input size=[4,1]; Ts parameter
function q_icrf2b_out  = fcn(omega_icrf2b,q_icrf2b, Ts)






w_cross = [  0   -omega_icrf2b(3)   omega_icrf2b(2);
            omega_icrf2b(3)    0   -omega_icrf2b(1);
           -omega_icrf2b(2)   omega_icrf2b(1)    0 ];

w_mat = [0        -omega_icrf2b';
         omega_icrf2b    -w_cross];


q_icrf2b_dot = 0.5 * w_mat * q_icrf2b;
q_icrf2b_out = q_icrf2b + q_icrf2b_dot * Ts;
% 
q_icrf2b_out = q_icrf2b_out / norm(q_icrf2b_out);
